simulink model "myexp6_3"  (R2022a)
settings: Solver=VariableStepAuto  StartTime=0.0  StopTime=100000  RelTol=1e-3
values from neighbouring files (symbols this model uses):
  A = 1    [exp6_2.m]
  k = k_list(i)    [exp6_2.m]
libraries: commsink2 x2, simulink x2, commutil2 x2, commchan3 x1, commrandsrc3 x1
settings Model: Creator=惠普  LastModifiedBy=惠普

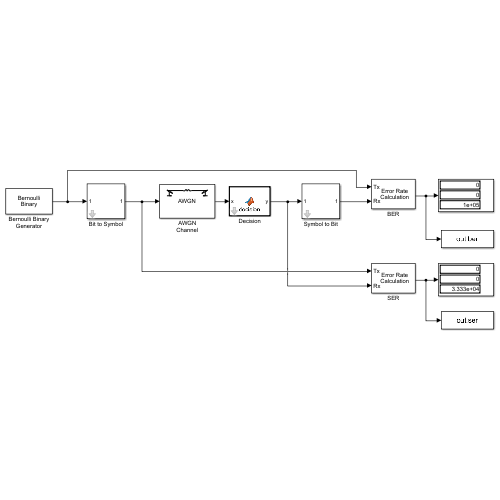
[thumbnail: Simulink's stored preview of the top-level diagram]
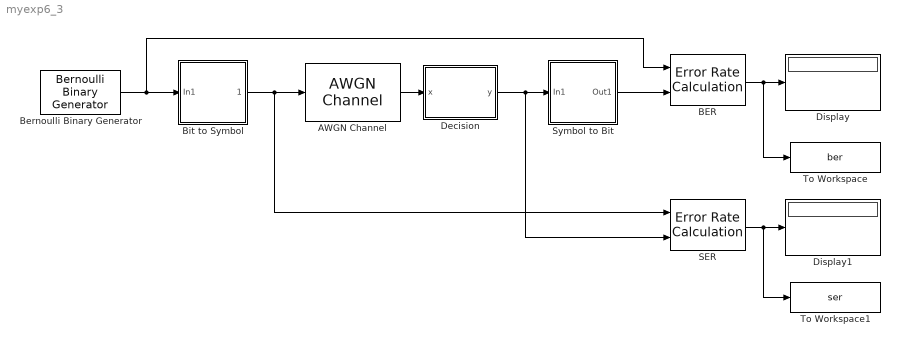
== system myexp6_3 ==
  AWGN Channel : commchan3/AWGN Channel  InputProcessing=Columns as channels (frame based)  seed=137  noiseMode=Variance from mask  EbNodB=10  EsNodB=10  SNRdB=10  bitsPerSym=1  Ps=1  Tsym=1  variance=sigma2
  BER : commsink2/Error Rate Calculation  N=(k>=2)*k  st_delay=0  cp_mode=Entire frame  subframe=[]  PMode=Port  WsName=ErrorVec  RsMode2=off  stop=off  numErr=100  maxBits=1e6
  Bernoulli Binary Generator : commrandsrc3/Bernoulli Binary Generator  ProbabilityOfZero=0.5  SeedSource=Auto  Seed=0  SampleTime=1  SamplesPerFrame=1  OutputDataType=double  SimulateUsing=Interpreted execution
  Bit to Symbol : Subsystem  mask(Bit to Symbol){k=k, A=A}
      mask prompts: k "Number of Bits"; A "Amplitude"
      mask DialogControl ParameterGroupVar Prompt: 参数
  Decision : MATLAB Function  TreatAsAtomicUnit=on  mask{k=k, A=A}
      mask prompts: k "Number of Bits"; A "Amplitude"
  Display : Display
  Display1 : Display
  SER : commsink2/Error Rate Calculation  N=0  st_delay=0  cp_mode=Entire frame  subframe=[]  PMode=Port  WsName=ErrorVec  RsMode2=off  stop=off  numErr=100  maxBits=1e6
  Symbol to Bit : Subsystem  mask(Symbol to Bit){k=k, A=A}
      mask prompts: k "Number of Bits"; A "Amplitude"
      mask DialogControl ParameterGroupVar Prompt: 参数
  To Workspace : ToWorkspace  VariableName=ber  SampleTime=-1
      settings: MaxDataPoints=1
  To Workspace1 : ToWorkspace  VariableName=ser  SampleTime=-1
      settings: MaxDataPoints=1
  wires:
  BER/1 -> To Workspace/1, Display/1
  Bit to Symbol/1(1) -> SER/1, AWGN Channel/1
  Bernoulli Binary Generator/1 -> BER/1, Bit to Symbol/1(In1)
  Symbol to Bit/1(Out1) -> BER/2
  SER/1 -> To Workspace1/1, Display1/1
  Decision/1(y) -> SER/2, Symbol to Bit/1(In1)
  AWGN Channel/1 -> Decision/1(x)

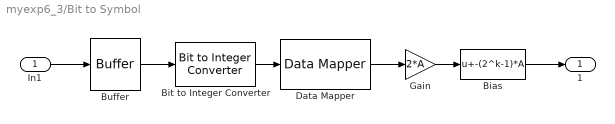
== system myexp6_3/Bit to Symbol ==
  In1 : Inport
  Bias : Bias  Bias=-(2^k-1)*A  SaturateOnIntegerOverflow=off
  Bit to Integer Converter : simulink/Logic and Bit Operations/Bit to Integer Converter  nbits=k  bitOrder=MSB first  signedOutputValues=Unsigned  outDtype=Inherit via internal rule  outDtypeSigned=Inherit via internal rule
      settings: SourceProductBaseCode=SL
  Buffer : Buffer  N=k  OutputFrames=off
  Data Mapper : commutil2/Data Mapper  MapMode=Binary to Gray  M=2^k  MapVec=[0 1 3 2 7 6 4 5]
      settings: SourceProductBaseCode=CM
  Gain : Gain  Gain=2*A
  1 : Outport
  wires:
  Gain/1 -> Bias/1
  Data Mapper/1 -> Gain/1
  Bit to Integer Converter/1 -> Data Mapper/1
  Bias/1 -> 1/1
  Buffer/1 -> Bit to Integer Converter/1
  In1/1 -> Buffer/1

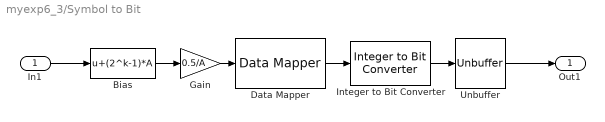
== system myexp6_3/Symbol to Bit ==
  In1 : Inport
  Bias : Bias  Bias=(2^k-1)*A  SaturateOnIntegerOverflow=off
  Data Mapper : commutil2/Data Mapper  MapMode=Gray to Binary  M=2^k  MapVec=[0 1 3 2 7 6 4 5]
      settings: SourceProductBaseCode=CM
  Gain : Gain  Gain=0.5/A
  Integer to Bit Converter : simulink/Logic and Bit Operations/Integer to Bit Converter  nbits=k  signedInputValues=Unsigned  bitOrder=MSB first  outDtype=Inherit via internal rule
      settings: SourceProductBaseCode=SL
  Unbuffer : Unbuffer
  Out1 : Outport
  wires:
  Data Mapper/1 -> Integer to Bit Converter/1
  Gain/1 -> Data Mapper/1
  In1/1 -> Bias/1
  Bias/1 -> Gain/1
  Integer to Bit Converter/1 -> Unbuffer/1
  Unbuffer/1 -> Out1/1

== matlab function myexp6_3/Decision ==
  data: x input; y output; A parameter; k parameter
function y = decision(x,A, k)
y = round((x+A)/(2*A))*2*A-A;
if (y < -(2^k-1)*A)
    y = -(2^k-1)*A;
elseif (y > (2^k-1)*A)
    y = (2^k-1)*A;
end
